simulink model "LLC_closed_loop_02"  (R2017b)
settings: Solver=VariableStepAuto  StartTime=0.0  StopTime=0.1  MaxStep=1e-4  RelTol=1e-4  EnableMultiTasking=on
PreLoadFcn:
  | Ts_Control=25e-6;
InitFcn:
  | Ts_Control=25e-6;
undefined symbols (not defined in the file): DiscIntNeverNeededParam
libraries: powerlib x18
Description:
  | Copyright 2008-2017 The MathWorks, Inc.
settings Model: Creator=MathWorks  LastModifiedBy=Saagar
settings SolverCC: SolverResetMethod=Robust
settings OptimizationCC: LifeSpan=inf
settings DebuggingCC: SFUnexpectedBacktrackingDiag=warning  SFNoUnconditionalDefaultTransitionDiag=warning  SFExecutionAtInitializationDiag=none
settings CodeAppCC: StateflowObjectComments=on
settings GRTTargetCC: TargetLangStandard=C89/C90 (ANSI)  GeneratePreprocessorConditionals=Disable all
settings ConfigComp: CovMetricSettings=dw  CovHtmlReporting=on  CovSaveCumulativeToWorkspaceVar=on  CovSaveSingleToWorkspaceVar=on  CovExternalEMLEnable=off
settings SimscapeCC: SimscapeNormalizeSystem=off

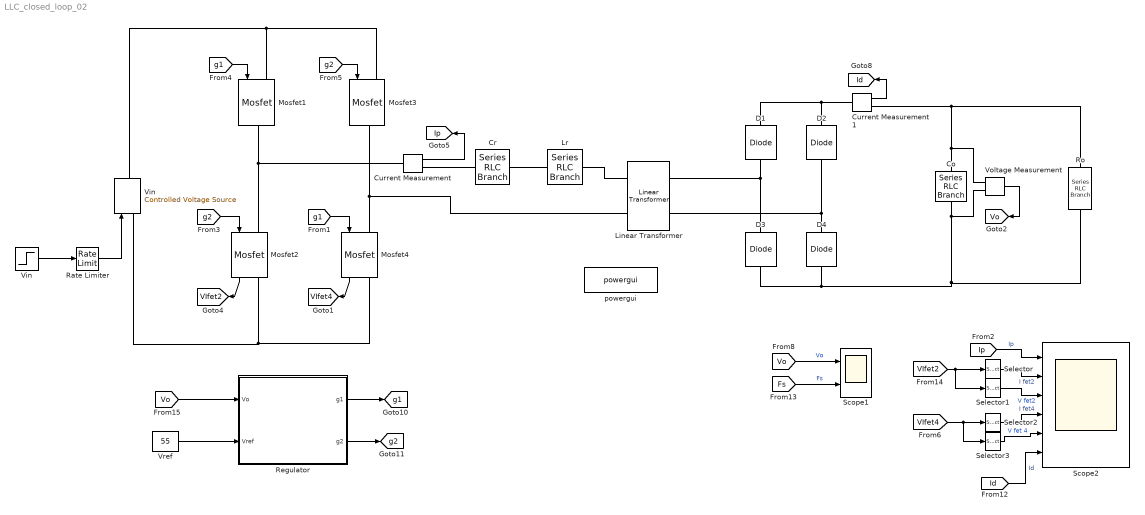
== system LLC_closed_loop_02 ==
  Co : powerlib/Elements/Series RLC Branch  LConnTagsString=__new0  RConnTagsString=__new0  BranchType=C  Resistance=1e-4  Inductance=200e-6  SetiL0=off  InitialCurrent=0  Capacitance=100e-6  Setx0=on  InitialVoltage=24  Measurements=None
  Cr : powerlib/Elements/Series RLC Branch  LConnTagsString=__new0  RConnTagsString=__new0  BranchType=C  Resistance=1e-4  Inductance=200e-6  SetiL0=off  InitialCurrent=0  Capacitance=160e-9  Setx0=off  InitialVoltage=40  Measurements=None
  Current Measurement : powerlib/Measurements/Current Measurement  PhasorSimulation=off  OutputType=Complex  PSBequivalent=0
  Current Measurement1 : powerlib/Measurements/Current Measurement  PhasorSimulation=off  OutputType=Complex  PSBequivalent=0
  D{1..4} (4 alike) : powerlib/Power Electronics/Diode  Ron=1e-3  Lon=0  Vf=0.5  IC=0  UseSnubber=off  Rs=1e6  Cs=inf  Measurements=off
  Linear Transformer : powerlib/Elements/Linear Transformer  UNITS=SI  NominalPower=[ 200 85e3 ]  winding1="[52   1e-2  75e-6]"  winding2="[6  1e-2  1.36e-6 ]"  ThreeWindings=off  winding3=[3.15e+05 0.7938 0.084225]  RmLm=[1e4 963e-6]  Measurements=None  DataType=on
  Lr : powerlib/Elements/Series RLC Branch  LConnTagsString=__new0  RConnTagsString=__new0  BranchType=L  Resistance=1e-4  Inductance=37.5e-6  SetiL0=off  InitialCurrent=0  Capacitance=15e-9  Setx0=off  InitialVoltage=40  Measurements=None
  Mosfet1 : powerlib/Power Electronics/Mosfet  Ron=1e-3  Lon=0  Rd=1e-3  Vfd=0  IC=0  Rs=1e6  Cs=inf  Measurements=off
  Mosfet2 : powerlib/Power Electronics/Mosfet  Ron=1e-3  Lon=0  Rd=1e-3  Vfd=0  IC=0  Rs=1e6  Cs=inf  Measurements=on
  Mosfet3 : powerlib/Power Electronics/Mosfet  Ron=1e-3  Lon=0  Rd=1e-3  Vfd=0  IC=0  Rs=1e6  Cs=inf  Measurements=off
  Mosfet4 : powerlib/Power Electronics/Mosfet  Ron=1e-3  Lon=0  Rd=1e-3  Vfd=0  IC=0  Rs=1e6  Cs=inf  Measurements=on
  Rate Limiter : RateLimiter  RisingSlewLimit=50e3  FallingSlewLimit=-50e3  SampleTimeMode=inherited  InitialCondition=390
  "Regulator " : Subsystem
  Ro : powerlib/Elements/Series RLC Branch  LConnTagsString=__new0  RConnTagsString=__new0  BranchType=R  Resistance=3  Inductance=200e-6  SetiL0=off  InitialCurrent=0  Capacitance=400e-6  Setx0=off  InitialVoltage=0  Measurements=None
  "Scope1 " : Scope  NumInputPorts=2
  Scope2 : Scope  NumInputPorts=6
  Selector : Selector  InputPortWidth=2  IndexOptions=Index vector (dialog)  Indices=1  OutputSizes=1
  Selector1 : Selector  InputPortWidth=2  IndexOptions=Index vector (dialog)  Indices=2  OutputSizes=1
  Selector2 : Selector  InputPortWidth=2  IndexOptions=Index vector (dialog)  Indices=1  OutputSizes=1
  Selector3 : Selector  InputPortWidth=2  IndexOptions=Index vector (dialog)  Indices=2  OutputSizes=1
  Vin : Step  Time=0.004  Before=320  After=320  SampleTime=Ts_Control
  "Vin " : powerlib/Electrical Sources/Controlled Voltage Source  Initialize=on  Source_Type=DC  Amplitude=0  Phase=0  Frequency=0  Measurements=None
  Voltage Measurement : powerlib/Measurements/Voltage Measurement  PhasorSimulation=off  OutputType=Complex  PSBequivalent=0
  Vref : Constant  Value=55
  powergui : powerlib/powergui  Priority=1  SimulationMode=Continuous  SampleTime=50e-6  frequency=60  Iterations=50  frequencyindice=0  Pbase=100e6  ErrMax=1e-4  UnitsV=kV  UnitsW=MW  buscounter=0  FunctionMessages=on  echomessages=off  EnableUseOfTLC=off  CurrentSourceSwitches=off  DisableSnubberDevices=off  DisableRonSwitches=off  DisableVfSwitches=off  DisplayEquations=off  SolverType=Tustin/Backward Euler (TBE)  Interpol=off  ExternalGateDelay=off  methode=off  Ts=100  x0status=blocks  SPID=on  SwTol=0  HookPort=off  RestoreLinks=warning  ResistiveCurrentMeasurement=off  Frange=[0:2:500]  Ylog=off  Xlog=on  ShowGrid=off  save=off  variable=ZData  structure=0  ZoomFFT=off  StartTime=0.0  cycles=1  DisplayStyle=1  fundamental=60  FreqAxis=off  MaxFrequency=1000  frequencyindicesteady=1  RmsSteady=1  display=off
  tag scope: Id=global, Ip=global, VIfet2=global, VIfet4=global, Vo=global, g1=global, g2=global
  wires:
  [g2] -> Mosfet2/1
  [g1] -> Mosfet1/1
  Current Measurement/1 -> [Ip]
  Voltage Measurement/1 -> [Vo]
  Current Measurement1/1 -> [Id]
  [VIfet2] -> Selector1/1, Selector/1
  [Vo] -> "Scope1 "/1  "Vo"
  Mosfet2/1 -> [VIfet2]
  Selector/1 -> Scope2/2  "I fet2"
  Selector1/1 -> Scope2/3  "V fet2"
  [Ip] -> Scope2/1  "Ip"
  Vin/1 -> Rate Limiter/1
  [Fs] -> "Scope1 "/2  "Fs"
  Rate Limiter/1 -> "Vin "/1
  [g1] -> Mosfet4/1
  [g2] -> Mosfet3/1
  Mosfet4/1 -> [VIfet4]
  [Vo] -> "Regulator "/1(Vo)
  Vref/1 -> "Regulator "/2(Vref)
  "Regulator "/1(g1) -> [g1]
  "Regulator "/2(g2) -> [g2]
  Selector2/1 -> Scope2/4  "I fet4"
  Selector3/1 -> Scope2/5  "V fet 4"
  [Id] -> Scope2/6  "Id"
  [VIfet4] -> Selector3/1, Selector2/1
  connections:
  Co/RConn1 -- Voltage Measurement/LConn2 -- Ro/RConn1 -- D4/LConn1 -- D3/LConn1
  Linear Transformer/RConn1 -- D3/RConn1 -- D1/LConn1
  Mosfet2/LConn1 -- Mosfet1/RConn1 -- Current Measurement/LConn1
  Linear Transformer/RConn2 -- D4/RConn1 -- D2/LConn1
  "Vin "/RConn1 -- Mosfet1/LConn1 -- Mosfet3/LConn1
  "Vin "/LConn1 -- Mosfet4/RConn1 -- Mosfet2/RConn1
  Cr/LConn1 -- Current Measurement/RConn1
  D1/RConn1 -- D2/RConn1 -- Current Measurement1/LConn1
  Voltage Measurement/LConn1 -- Ro/LConn1 -- Current Measurement1/RConn1 -- Co/LConn1
  Mosfet4/LConn1 -- Linear Transformer/LConn2 -- Mosfet3/RConn1
  Lr/LConn1 -- Cr/RConn1
  Lr/RConn1 -- Linear Transformer/LConn1

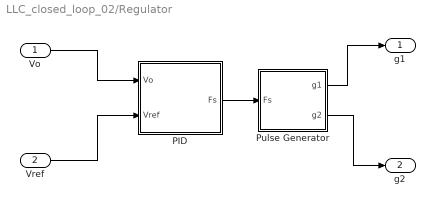
== system LLC_closed_loop_02/Regulator  ==
  Vo : Inport
  Vref : Inport  Port=2
  PID : Subsystem
  Pulse Generator : Subsystem
  g1 : Outport
  g2 : Outport  Port=2
  wires:
  Vref/1 -> PID/2(Vref)
  Vo/1 -> PID/1(Vo)
  Pulse Generator/1(g1) -> g1/1
  Pulse Generator/2(g2) -> g2/1
  PID/1(Fs) -> Pulse Generator/1(Fs)

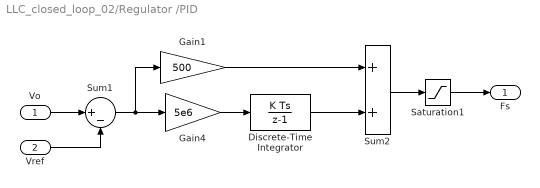
== system LLC_closed_loop_02/Regulator /PID ==
  Vo : Inport
  Vref : Inport  Port=2
  Discrete-Time Integrator : DiscreteIntegrator  InitialCondition=91.2e3  InitialConditionSetting=State (most efficient)  SampleTime=Ts_Control  LimitOutput=on  UpperSaturationLimit=300e3  LowerSaturationLimit=10e3  ICPrevOutput=DiscIntNeverNeededParam  ICPrevScaledInput=DiscIntNeverNeededParam
  Gain1 : Gain  Gain=500  SaturateOnIntegerOverflow=on  OutDataTypeStr=Inherit: Same as input  ParamDataTypeStr=Inherit: Same as input
  Gain4 : Gain  Gain=5e6  SaturateOnIntegerOverflow=on  OutDataTypeStr=Inherit: Same as input  ParamDataTypeStr=Inherit: Same as input
  Saturation1 : Saturate  UpperLimit=300e3  LowerLimit=10e3
  Sum1 : Sum  Inputs=|+-  SaturateOnIntegerOverflow=on  InputSameDT=on  OutDataTypeStr=Inherit: Same as first input
  Sum2 : Sum  SaturateOnIntegerOverflow=on  InputSameDT=on  OutDataTypeStr=Inherit: Same as first input
  Fs : Outport
  wires:
  Vo/1 -> Sum1/1
  Vref/1 -> Sum1/2
  Sum1/1 -> Gain1/1, Gain4/1
  Gain4/1 -> Discrete-Time Integrator/1
  Discrete-Time Integrator/1 -> Sum2/2
  Sum2/1 -> Saturation1/1
  Gain1/1 -> Sum2/1
  Saturation1/1 -> Fs/1

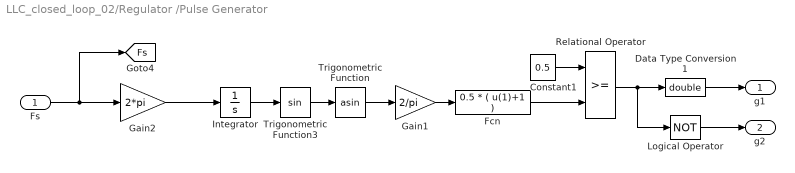
== system LLC_closed_loop_02/Regulator /Pulse Generator ==
  Fs : Inport
  Constant1 : Constant  Value=0.5
  Data Type Conversion1 : DataTypeConversion  OutDataTypeStr=double
  Fcn : Fcn  Expr=0.5 * ( u(1)+1 )
  Gain1 : Gain  Gain=2/pi  SaturateOnIntegerOverflow=on  OutDataTypeStr=Inherit: Same as input  ParamDataTypeStr=Inherit: Same as input
  Gain2 : Gain  Gain=2*pi  SaturateOnIntegerOverflow=on  OutDataTypeStr=Inherit: Same as input  ParamDataTypeStr=Inherit: Same as input
  Integrator : Integrator
  Logical Operator : Logic  Operator=NOT  AllPortsSameDT=off  OutDataTypeStr=float('double')
  Relational Operator : RelationalOperator  OutDataTypeStr=boolean  RndMeth=Nearest
  Trigonometric Function : Trigonometry  Operator=asin
  Trigonometric Function3 : Trigonometry
  g1 : Outport
  g2 : Outport  Port=2
  tag scope: Fs=global
  wires:
  Fs/1 -> Gain2/1, [Fs]
  Gain2/1 -> Integrator/1
  Data Type Conversion1/1 -> g1/1
  Logical Operator/1 -> g2/1
  Fcn/1 -> Relational Operator/2
  Relational Operator/1 -> Logical Operator/1, Data Type Conversion1/1
  Constant1/1 -> Relational Operator/1
  Integrator/1 -> Trigonometric Function3/1
  Trigonometric Function/1 -> Gain1/1
  Gain1/1 -> Fcn/1
  Trigonometric Function3/1 -> Trigonometric Function/1
